simulink model "model_float"  (R2022a)
settings: Solver=FixedStepAuto  StartTime=0.0  StopTime=1e2  RelTol=1e-3
settings Model: Creator=mrem  LastModifiedBy=mrem

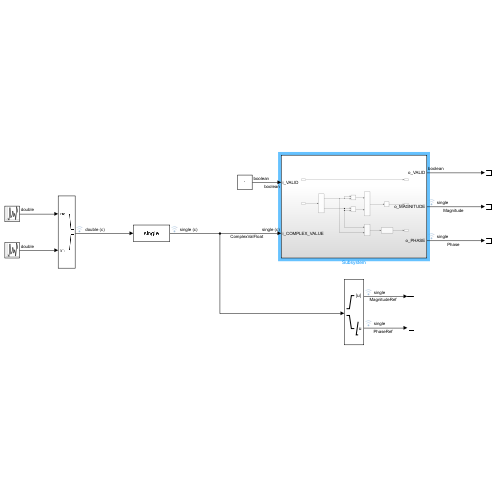
[thumbnail: Simulink's stored preview of the top-level diagram]
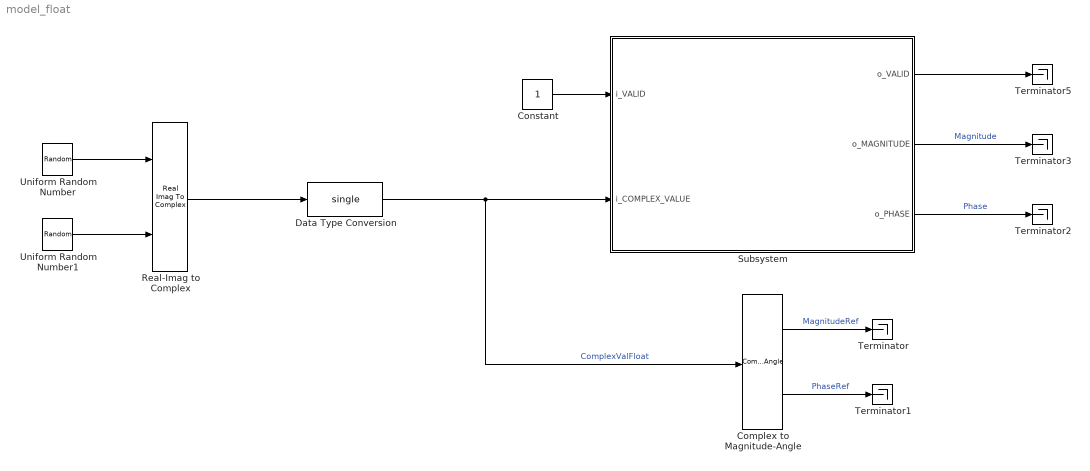
== system model_float ==
  Complex to Magnitude-Angle : ComplexToMagnitudeAngle
  Constant : Constant  OutDataTypeStr=boolean  SampleTime=-1
  Data Type Conversion : DataTypeConversion  OutDataTypeStr=single  RndMeth=Round  SaturateOnIntegerOverflow=off
  Real-Imag to Complex : RealImagToComplex
  Subsystem : Subsystem
  Terminator{,1..3,5} (5 alike) : Terminator
  Uniform Random Number : UniformRandomNumber  Minimum=0  Maximum=16777215.9909375  Seed=24  SampleTime=1
  Uniform Random Number1 : UniformRandomNumber  Minimum=0  Maximum=16777215.9909375  Seed=25  SampleTime=1
  wires:
  Complex to Magnitude-Angle/1 -> Terminator/1  "MagnitudeRef"
  Data Type Conversion/1 -> Complex to Magnitude-Angle/1, Subsystem/2(i_COMPLEX_VALUE)  "ComplexValFloat"
  Subsystem/1(o_VALID) -> Terminator5/1
  Complex to Magnitude-Angle/2 -> Terminator1/1  "PhaseRef"
  Uniform Random Number1/1 -> Real-Imag to Complex/2
  Real-Imag to Complex/1 -> Data Type Conversion/1
  Uniform Random Number/1 -> Real-Imag to Complex/1
  Subsystem/3(o_PHASE) -> Terminator2/1  "Phase"
  Subsystem/2(o_MAGNITUDE) -> Terminator3/1  "Magnitude"
  Constant/1 -> Subsystem/1(i_VALID)

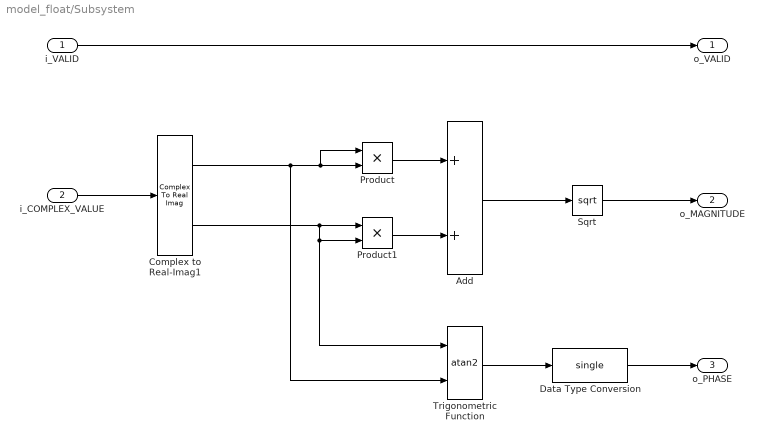
== system model_float/Subsystem ==
  i_VALID : Inport  OutDataTypeStr=boolean
  i_COMPLEX_VALUE : Inport  Port=2  OutDataTypeStr=single  LockScale=on
      settings: SignalType=complex
  Add : Sum
  Complex to Real-Imag1 : ComplexToRealImag
  Data Type Conversion : DataTypeConversion  OutDataTypeStr=single  SaturateOnIntegerOverflow=off  RndMeth=Floor
  Product : Product
  Product1 : Product
  Sqrt : Sqrt  OutDataTypeStr=single
  Trigonometric Function : Trigonometry  Operator=atan2
  o_VALID : Outport  OutDataTypeStr=boolean
  o_MAGNITUDE : Outport  Port=2
  o_PHASE : Outport  Port=3
  wires:
  Complex to Real-Imag1/1 -> Trigonometric Function/2, Product/1, Product/2
  Complex to Real-Imag1/2 -> Trigonometric Function/1, Product1/2, Product1/1
  Product/1 -> Add/1
  Product1/1 -> Add/2
  Add/1 -> Sqrt/1
  Sqrt/1 -> o_MAGNITUDE/1
  i_COMPLEX_VALUE/1 -> Complex to Real-Imag1/1
  Trigonometric Function/1 -> Data Type Conversion/1
  Data Type Conversion/1 -> o_PHASE/1
  i_VALID/1 -> o_VALID/1
